simulink model "MODELODETURBINADERIO2017a"  (R2017a)
settings: Solver=FixedStepAuto  StartTime=0.0  StopTime=500  FixedStep=50e-3  RelTol=1e-3
values from neighbouring files (symbols this model uses):
  A = pi()*((D/2)^2)    [MODELOHIDRO.m]    (also in MODELOHIDROV10.m; MODELOHIDROV2.m; MODELOHIDROV3.m; MODELOHIDROV4.m)
  a = 790.51    [MODELOHIDRO.m]    (also in MODELOHIDROV2.m; MODELOHIDROV3.m)
  B = 0    [MODELOHIDRO.m]    (also in MODELOHIDROV10.m; MODELOHIDROV2.m; MODELOHIDROV3.m; MODELOHIDROV4.m)
  b = 6900.50    (= 6900.5)    [MODELOHIDRO.m]    (also in MODELOHIDROV2.m; MODELOHIDROV3.m)
  Bi = 0.2287    [MODELOHIDRO.m]    (also in MODELOHIDROV10.m = 0.1; MODELOHIDROV2.m; MODELOHIDROV3.m; MODELOHIDROV4.m = 0.005)
  c = 23794    [MODELOHIDRO.m]    (also in MODELOHIDROV2.m; MODELOHIDROV3.m)
  D = 1    [MODELOHIDRO.m]    (also in MODELOHIDROV10.m; MODELOHIDROV2.m; MODELOHIDROV3.m; MODELOHIDROV4.m)
  d = 39268    [MODELOHIDRO.m]    (also in MODELOHIDROV2.m; MODELOHIDROV3.m)
  den = 1000    [MODELOHIDRO.m]    (also in MODELOHIDROV10.m; MODELOHIDROV2.m; MODELOHIDROV3.m; MODELOHIDROV4.m)
  e = 31863    [MODELOHIDRO.m]    (also in MODELOHIDROV2.m; MODELOHIDROV3.m)
  f = 10049    [MODELOHIDRO.m]    (also in MODELOHIDROV2.m; MODELOHIDROV3.m)
  FACTOR = 1/(2*pi())*60    [MODELOHIDRO.m]    (also in MODELOHIDROV2.m; MODELOHIDROV3.m)
  Ji = 1    [MODELOHIDRO.m]    (also in MODELOHIDROV10.m = 1.72; MODELOHIDROV2.m; MODELOHIDROV3.m; MODELOHIDROV4.m = 0.0465)
  k = 1    [MODELOHIDRO.m]    (also in MODELOHIDROV2.m; MODELOHIDROV3.m)
  Kb = 1.8    [MODELOHIDRO.m]    (also in MODELOHIDROV10.m = 6.2; MODELOHIDROV2.m; MODELOHIDROV3.m; MODELOHIDROV4.m = 0.027)
  Kp = 0.4    [MODELOHIDRO.m]    (also in MODELOHIDROV10.m = 5.6627; MODELOHIDROV2.m; MODELOHIDROV3.m; MODELOHIDROV4.m = 0.027)
  m = 5    [MODELOHIDRO.m]    (also in MODELOHIDROV2.m; MODELOHIDROV3.m)
  r = D/2    (= 0.5)    [MODELOHIDRO.m]    (also in MODELOHIDROV10.m; MODELOHIDROV2.m; MODELOHIDROV3.m; MODELOHIDROV4.m)
  Ri = 0.6    [MODELOHIDRO.m]    (also in MODELOHIDROV10.m = 0.973; MODELOHIDROV2.m; MODELOHIDROV3.m; MODELOHIDROV4.m = 1)
  T_d = 0    [MODELOHIDRO.m]    (also in MODELOHIDROV10.m; MODELOHIDROV2.m; MODELOHIDROV3.m; MODELOHIDROV4.m)
  z = 2    [MODELOHIDRO.m]    (also in MODELOHIDROV2.m; MODELOHIDROV3.m)
undefined symbols (not defined in the file or in its folder): sigbuilder_block
libraries: simulink x3
settings Model: Creator=zni.uao  LastModifiedBy=Hp 14
settings SimscapeCC: SimscapeNormalizeSystem=off

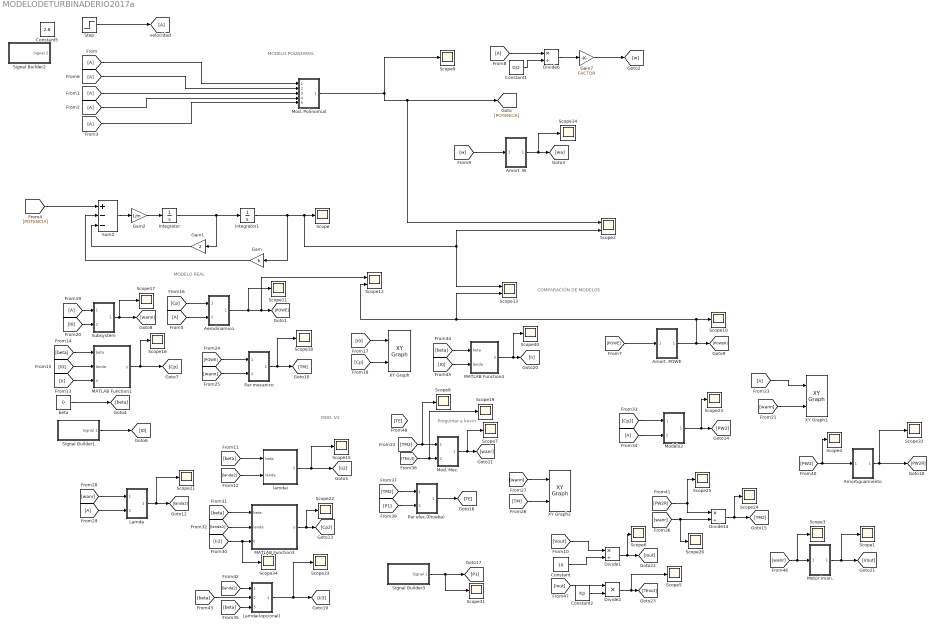
== system MODELODETURBINADERIO2017a ==
  note: MODELO POLINOMIAL
  note: MODELO REAL
  note: COMPARACIÓN DE MODELOS
  note: MOD. V2
  note: Preguntar a kevin
  Aerodinamico : Subsystem
  Amort. POWE : Subsystem
  Amort. W : Subsystem
  Amortiguamiento : Subsystem
  Constant : Constant  Value=10
  Constant1 : Constant  Value=D/2
  Constant2 : Constant  Value=Kp
  Constant5 : Constant  Value=2.8
  Divide1 : Product  Inputs=*/
  Divide14 : Product  Inputs=*/
  Divide2 : Product  Inputs=**
  Divide6 : Product  Inputs=*/
  Gain : Gain  Gain=k
  Gain1 : Gain  Gain=z
  Gain2 : Gain  Gain=1/m
  Gain7 : Gain  Gain=FACTOR
  Integrator : Integrator
  Integrator1 : Integrator
  Lamda : Subsystem
  Lamdai(opcional) : Subsystem
  MATLAB Function1 : MATLAB Function  TreatAsAtomicUnit=on
  MATLAB Function3 : MATLAB Function  TreatAsAtomicUnit=on
  MATLAB Function4 : MATLAB Function  TreatAsAtomicUnit=on
  Mod. Mec. : Subsystem
  Mod. Polinomial : Subsystem
  Modelo2 : Subsystem
  Motor iman. : Subsystem
  Par elec.(Prueba) : Subsystem
  Par mecanico : Subsystem
  Scope{,1,3..11,14..19,21..26,31..34,40} (28 alike) : Scope
  Scope12 : Scope  NumInputPorts=2
  Scope13 : Scope  NumInputPorts=2
  Scope2 : Scope  NumInputPorts=2
  Signal Builder1 : Subsystem  Tag=STV Subsys  LoadFcn=sigbuilder_block('load');  StartFcn=sigbuilder_block('start');  StopFcn=sigbuilder_block('stop');  ClipboardFcn=sigbuilder_block('clipboard');  mask(Sigbuilder block){tuvar=[0:10]}
      mask help: Simulink:masks:SigbuilderBlock_MD
      mask init:
      | if ~strcmp(get_param(bdroot(gcbh),'SimulationStatus'),'stopped') tuvar = sigbuilder_block('maskInit'); end
      settings: CopyFcn=sigbuilder_block('copy');  DeleteFcn=sigbuilder_block('delete');  ModelCloseFcn=sigbuilder_block('modelClose');  PreSaveFcn=sigbuilder_block('preSave');  PauseFcn=sigbuilder_block('pause');  ContinueFcn=sigbuilder_block('continue');  NameChangeFcn=sigbuilder_block('namechange');  OpenFcn=sigbuilder_block('open',[169.5 67.5 550.5 359.25 ]);  CloseFcn=sigbuilder_block('close');
      mask Display: plot(0, 0, 100, 100,[2, 2, 32, 32, 2], [68, 8, 8, 68, 68],[32, 2], [38, 38], [32, 19, 2],[53, 60, 44], [32, 17, 17, 2],[16, 16, 31, 31]);txt = getActiveGroup(gcbh);text(2, 100, txt,'verticalAlignment', 'top');
  Signal Builder2 : Subsystem  Tag=STV Subsys  LoadFcn=sigbuilder_block('load');  StartFcn=sigbuilder_block('start');  StopFcn=sigbuilder_block('stop');  ClipboardFcn=sigbuilder_block('clipboard');  mask(Sigbuilder block){tuvar=[0:10]}
      mask help: Simulink:masks:SigbuilderBlock_MD
      mask init:
      | if ~strcmp(get_param(bdroot(gcbh),'SimulationStatus'),'stopped') tuvar = sigbuilder_block('maskInit'); end
      settings: CopyFcn=sigbuilder_block('copy');  DeleteFcn=sigbuilder_block('delete');  ModelCloseFcn=sigbuilder_block('modelClose');  PreSaveFcn=sigbuilder_block('preSave');  PauseFcn=sigbuilder_block('pause');  ContinueFcn=sigbuilder_block('continue');  NameChangeFcn=sigbuilder_block('namechange');  OpenFcn=sigbuilder_block('open',[197.25 66 550.5 359.25 ]);  CloseFcn=sigbuilder_block('close');
      mask Display: plot(0, 0, 100, 100,[2, 2, 32, 32, 2], [68, 8, 8, 68, 68],[32, 2], [38, 38], [32, 19, 2],[53, 60, 44], [32, 17, 17, 2],[16, 16, 31, 31]);txt = getActiveGroup(gcbh);text(2, 100, txt,'verticalAlignment', 'top');
  Signal Builder3 : Subsystem  Tag=STV Subsys  LoadFcn=sigbuilder_block('load');  StartFcn=sigbuilder_block('start');  StopFcn=sigbuilder_block('stop');  ClipboardFcn=sigbuilder_block('clipboard');  mask(Sigbuilder block){tuvar=[0:10]}
      mask help: Simulink:masks:SigbuilderBlock_MD
      mask init:
      | if ~strcmp(get_param(bdroot(gcbh),'SimulationStatus'),'stopped') tuvar = sigbuilder_block('maskInit'); end
      settings: CopyFcn=sigbuilder_block('copy');  DeleteFcn=sigbuilder_block('delete');  ModelCloseFcn=sigbuilder_block('modelClose');  PreSaveFcn=sigbuilder_block('preSave');  PauseFcn=sigbuilder_block('pause');  ContinueFcn=sigbuilder_block('continue');  NameChangeFcn=sigbuilder_block('namechange');  OpenFcn=sigbuilder_block('open',[250.5 81.75 550.5 359.25 ]);  CloseFcn=sigbuilder_block('close');
      mask Display: plot(0, 0, 100, 100,[2, 2, 32, 32, 2], [68, 8, 8, 68, 68],[32, 2], [38, 38], [32, 19, 2],[53, 60, 44], [32, 17, 17, 2],[16, 16, 31, 31]);txt = getActiveGroup(gcbh);text(2, 100, txt,'verticalAlignment', 'top');
  Step : Step  Time=250  Before=2.5  After=2.888  SampleTime=0
  Subsystem : Subsystem
  Sum2 : Sum  Inputs=+--
  XY Graph : simulink/Sinks/XY Graph  xmin=1  xmax=20  ymin=0  ymax=0.56  st=0.1
  XY Graph1 : simulink/Sinks/XY Graph  xmin=1  xmax=20  ymin=0  ymax=0.56  st=0.1
  XY Graph2 : simulink/Sinks/XY Graph  xmin=1  xmax=20  ymin=0  ymax=0.56  st=0.1
  beta : Constant  Value=0
  lamdai : MATLAB Function  TreatAsAtomicUnit=on
  wires:
  Gain/1 -> Sum2/2
  Integrator1/1 -> Scope13/1, Scope2/2, Scope/1, Gain/1
  Gain1/1 -> Sum2/3
  Sum2/1 -> Gain2/1
  Gain2/1 -> Integrator/1
  [POTENCIA] -> Sum2/1
  Integrator/1 -> Gain1/1, Integrator1/1
  [A] -> Divide6/1
  Constant1/1 -> Divide6/2
  Divide6/1 -> Gain7/1
  Gain7/1 -> [w]
  beta/1 -> [beta]
  [Ii] -> MATLAB Function1/3(Ii)
  [beta] -> MATLAB Function1/1(beta)
  [I0] -> MATLAB Function1/2(landa)
  MATLAB Function1/1(y) -> Scope16/1, [Cp]
  [I0] -> XY Graph/1
  [wann] -> XY Graph1/2
  [A] -> XY Graph1/1
  [TM] -> XY Graph2/2
  [wann] -> XY Graph2/1
  MATLAB Function3/1(y) -> [Cp2], Scope22/1
  [beta] -> MATLAB Function3/1(beta)
  [landa2] -> MATLAB Function3/2(landa)
  [Ii2] -> Scope34/1, MATLAB Function3/3(Ii)
  Divide14/1 -> [TM2], Scope24/1
  [wanr] -> Scope26/1, Divide14/2
  [PW2R] -> Scope25/1, Divide14/1
  Signal Builder3/1(Signal 1) -> Scope31/1, [P1]
  [PW2] -> Amortiguamiento/1(In1), Scope4/1
  MATLAB Function4/1(Ii) -> Scope40/1, [Ii]
  [I0] -> MATLAB Function4/2(landa)
  [beta] -> MATLAB Function4/1(beta)
  lamdai/1(Ii) -> [Ii2], Scope15/1
  [landa2] -> lamdai/2(landa)
  [beta] -> lamdai/1(beta)
  Signal Builder1/1(Signal 1) -> [I0]
  Modelo2/1(Out1) -> Scope23/1, [PW2]
  [Cp2] -> Modelo2/1(In1)
  [A] -> Modelo2/2(In2)
  Par mecanico/1(Out1) -> [TM], Scope18/1
  [POWE] -> Par mecanico/1(In1)
  [wann] -> Par mecanico/2(In2)
  Aerodinamico/1(Out1) -> Scope11/1, Scope12/1, [POWE]
  [Cp] -> Aerodinamico/1(In1)
  [A] -> Aerodinamico/2(In2)
  [TM2] -> Par elec.(Prueba)/1(In1)
  [P1] -> Par elec.(Prueba)/2(In2)
  Par elec.(Prueba)/1(Out1) -> [TE]
  Lamda/1(Out1) -> [landa2], Scope21/1
  [wanr] -> Lamda/1(In1)
  [A] -> Lamda/2(In2)
  Lamdai(opcional)/1(Out1) -> Scope33/1, [Ii3]
  [landa2] -> Lamdai(opcional)/1(In1)
  [beta] -> Lamdai(opcional)/2(In2)
  [beta] -> Lamdai(opcional)/3(In3)
  [TM2] -> Scope8/1, Mod. Mec./1(In1)
  [TEout] -> Scope19/1, Mod. Mec./2(In2)
  Mod. Mec./1(Out1) -> Scope7/1, [wanr]
  [Cp] -> XY Graph/2
  Mod. Polinomial/1(Out1) -> Scope2/1, [POTENCIA], Scope9/1
  [A] -> Mod. Polinomial/1(In1)
  [A] -> Mod. Polinomial/2(In2)
  [A] -> Mod. Polinomial/3(In3)
  [A] -> Mod. Polinomial/4(In4)
  [A] -> Mod. Polinomial/5(In5)
  [wanr] -> Scope3/1, Motor iman./1(In1)
  Motor iman./1(Out1) -> Scope1/1, [Vout]
  Amortiguamiento/1(Out1) -> Scope32/1, [PW2R]
  Subsystem/1(Out1) -> [wann], Scope17/1
  [A] -> Subsystem/1(In1)
  [I0] -> Subsystem/2(In2)
  Amort. POWE/1(Out1) -> [POWER], Scope10/1, Scope12/2, Scope13/2
  [POWE] -> Amort. POWE/1(In1)
  [w] -> Amort. W/1(In1)
  Amort. W/1(Out1) -> Scope14/1, [wa]
  [Vout] -> Divide1/1
  Constant/1 -> Divide1/2
  Divide1/1 -> Scope6/1, [Iout]
  [Iout] -> Divide2/1
  Constant2/1 -> Divide2/2
  Divide2/1 -> Scope5/1, [TEout]
  Step/1 -> [A]

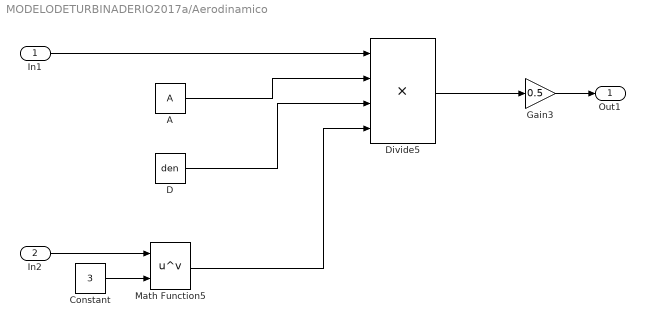
== system MODELODETURBINADERIO2017a/Aerodinamico ==
  In1 : Inport
  In2 : Inport  Port=2
  A : Constant  Value=A
  Constant : Constant  Value=3
  D : Constant  Value=den
  Divide5 : Product  Inputs=****  SaturateOnIntegerOverflow=on  RndMeth=Zero
  Gain3 : Gain  Gain=0.5
  Math Function5 : Math  Operator=pow  SaturateOnIntegerOverflow=on
  Out1 : Outport
  wires:
  Constant/1 -> Math Function5/2
  In2/1 -> Math Function5/1
  Math Function5/1 -> Divide5/4
  A/1 -> Divide5/2
  Divide5/1 -> Gain3/1
  D/1 -> Divide5/3
  In1/1 -> Divide5/1
  Gain3/1 -> Out1/1

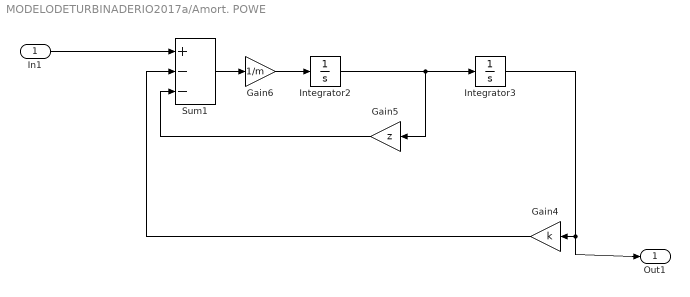
== system MODELODETURBINADERIO2017a/Amort. POWE ==
  In1 : Inport
  Gain4 : Gain  Gain=k
  Gain5 : Gain  Gain=z
  Gain6 : Gain  Gain=1/m
  Integrator2 : Integrator
  Integrator3 : Integrator
  Sum1 : Sum  Inputs=+--
  Out1 : Outport
  wires:
  Sum1/1 -> Gain6/1
  Integrator3/1 -> Out1/1, Gain4/1
  Gain4/1 -> Sum1/2
  Integrator2/1 -> Gain5/1, Integrator3/1
  Gain5/1 -> Sum1/3
  In1/1 -> Sum1/1
  Gain6/1 -> Integrator2/1

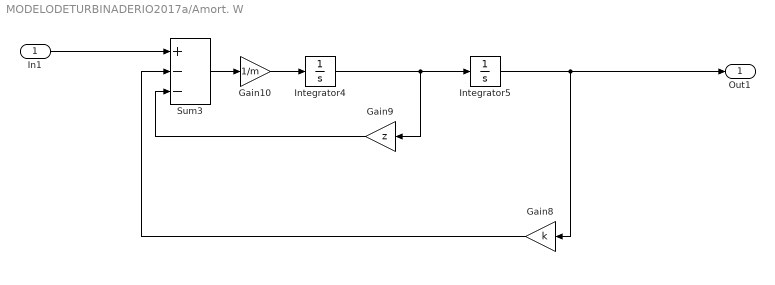
== system MODELODETURBINADERIO2017a/Amort. W ==
  In1 : Inport
  Gain10 : Gain  Gain=1/m
  Gain8 : Gain  Gain=k
  Gain9 : Gain  Gain=z
  Integrator4 : Integrator
  Integrator5 : Integrator
  Sum3 : Sum  Inputs=+--
  Out1 : Outport
  wires:
  In1/1 -> Sum3/1
  Gain9/1 -> Sum3/3
  Integrator4/1 -> Gain9/1, Integrator5/1
  Sum3/1 -> Gain10/1
  Integrator5/1 -> Out1/1, Gain8/1
  Gain10/1 -> Integrator4/1
  Gain8/1 -> Sum3/2

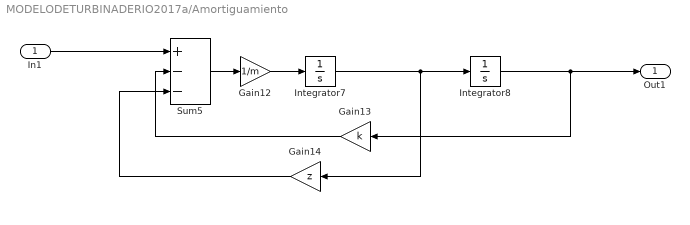
== system MODELODETURBINADERIO2017a/Amortiguamiento ==
  In1 : Inport
  Gain12 : Gain  Gain=1/m
  Gain13 : Gain  Gain=k
  Gain14 : Gain  Gain=z
  Integrator7 : Integrator
  Integrator8 : Integrator
  Sum5 : Sum  Inputs=+--
  Out1 : Outport
  wires:
  Gain13/1 -> Sum5/2
  Integrator8/1 -> Out1/1, Gain13/1
  Integrator7/1 -> Gain14/1, Integrator8/1
  Sum5/1 -> Gain12/1
  Gain12/1 -> Integrator7/1
  Gain14/1 -> Sum5/3
  In1/1 -> Sum5/1

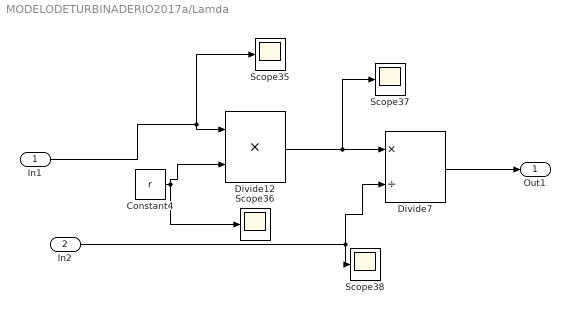
== system MODELODETURBINADERIO2017a/Lamda ==
  In1 : Inport
  In2 : Inport  Port=2
  Constant4 : Constant  Value=r
  Divide12 : Product  Inputs=**
  Divide7 : Product  Inputs=*/
  Scope{35..38} (4 alike) : Scope
  Out1 : Outport
  wires:
  Divide7/1 -> Out1/1
  In1/1 -> Divide12/1, Scope35/1
  Constant4/1 -> Divide12/2, Scope36/1
  In2/1 -> Divide7/2, Scope38/1
  Divide12/1 -> Scope37/1, Divide7/1

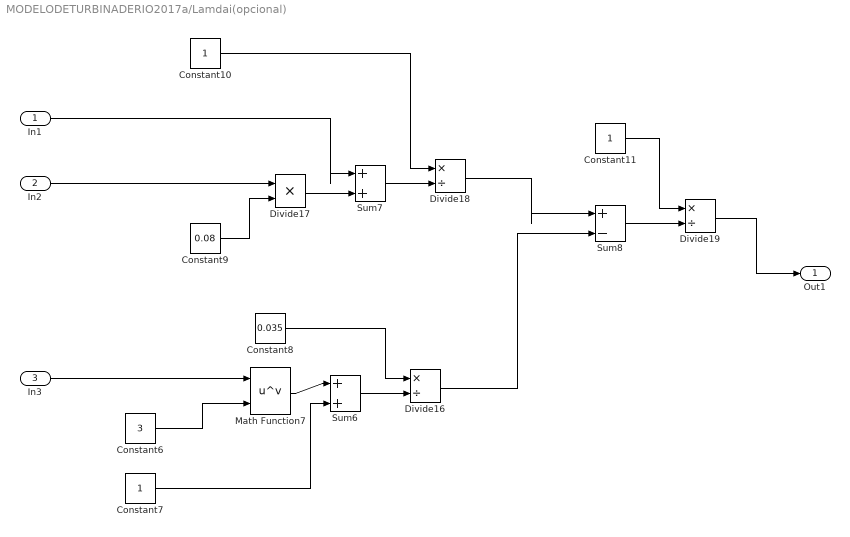
== system MODELODETURBINADERIO2017a/Lamdai(opcional) ==
  In1 : Inport
  In2 : Inport  Port=2
  In3 : Inport  Port=3
  Constant10 : Constant
  Constant11 : Constant
  Constant6 : Constant  Value=3
  Constant7 : Constant
  Constant8 : Constant  Value=0.035
  Constant9 : Constant  Value=0.08
  Divide16 : Product  Inputs=*/  SaturateOnIntegerOverflow=on  RndMeth=Zero
  Divide17 : Product  Inputs=**  SaturateOnIntegerOverflow=on  RndMeth=Zero
  Divide18 : Product  Inputs=*/  SaturateOnIntegerOverflow=on  RndMeth=Zero
  Divide19 : Product  Inputs=*/  SaturateOnIntegerOverflow=on  RndMeth=Zero
  Math Function7 : Math  Operator=pow  SaturateOnIntegerOverflow=on
  Sum6 : Sum  Inputs=|++
  Sum7 : Sum  Inputs=|++
  Sum8 : Sum  Inputs=|+-
  Out1 : Outport
  wires:
  Divide19/1 -> Out1/1
  Constant6/1 -> Math Function7/2
  Math Function7/1 -> Sum6/1
  Constant7/1 -> Sum6/2
  Sum6/1 -> Divide16/2
  In2/1 -> Divide17/1
  Constant8/1 -> Divide16/1
  Constant9/1 -> Divide17/2
  Divide17/1 -> Sum7/2
  In1/1 -> Sum7/1
  In3/1 -> Math Function7/1
  Sum8/1 -> Divide19/2
  Constant11/1 -> Divide19/1
  Constant10/1 -> Divide18/1
  Divide18/1 -> Sum8/1
  Sum7/1 -> Divide18/2
  Divide16/1 -> Sum8/2

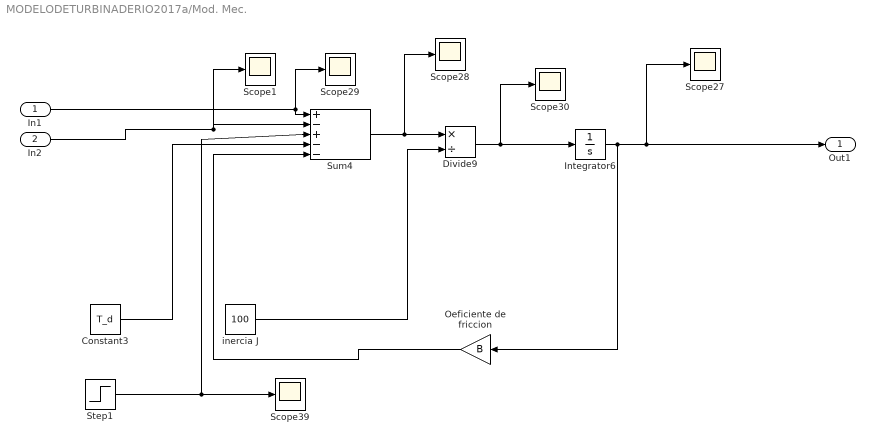
== system MODELODETURBINADERIO2017a/Mod. Mec. ==
  In1 : Inport
  In2 : Inport  Port=2
  Constant3 : Constant  Value=T_d
  Divide9 : Product  Inputs=*/
  Integrator6 : Integrator  InitialCondition=10
  Oeficiente de friccion : Gain  Gain=B
  Scope{1,27..30,39} (6 alike) : Scope
  Step1 : Step  Time=3  Before=5  After=0  SampleTime=0
  Sum4 : Sum  Inputs=|+-+--
  inercia J : Constant  Value=100
  Out1 : Outport
  wires:
  Oeficiente de friccion/1 -> Sum4/5
  Constant3/1 -> Sum4/4
  In2/1 -> Scope1/1, Sum4/2
  inercia J/1 -> Divide9/2
  Divide9/1 -> Scope30/1, Integrator6/1
  Sum4/1 -> Scope28/1, Divide9/1
  Integrator6/1 -> Out1/1, Scope27/1, Oeficiente de friccion/1
  In1/1 -> Scope29/1, Sum4/1
  Step1/1 -> Scope39/1, Sum4/3

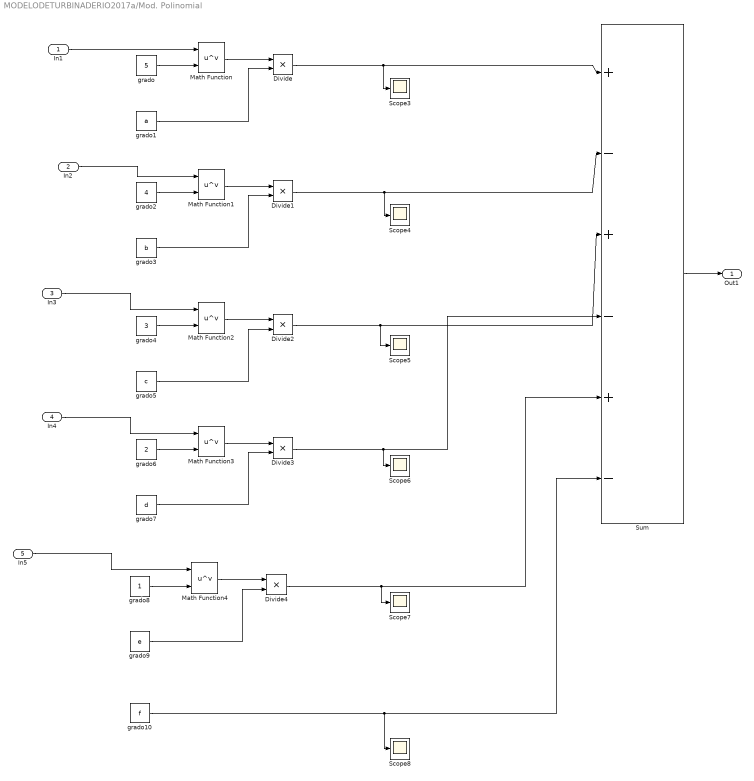
== system MODELODETURBINADERIO2017a/Mod. Polinomial ==
  In1 : Inport
  In2 : Inport  Port=2
  In3 : Inport  Port=3
  In4 : Inport  Port=4
  In5 : Inport  Port=5
  Divide{,1..4} (5 alike) : Product  Inputs=**
  Math Function{,1..4} (5 alike) : Math  Operator=pow  SaturateOnIntegerOverflow=on
  Scope{3..8} (6 alike) : Scope
  Sum : Sum  Inputs=|+-+-+-
  grado : Constant  Value=5
  grado1 : Constant  Value=a
  grado10 : Constant  Value=f
  grado2 : Constant  Value=4
  grado3 : Constant  Value=b
  grado4 : Constant  Value=3
  grado5 : Constant  Value=c
  grado6 : Constant  Value=2
  grado7 : Constant  Value=d
  grado8 : Constant
  grado9 : Constant  Value=e
  Out1 : Outport
  wires:
  In3/1 -> Math Function2/1
  Sum/1 -> Out1/1
  grado/1 -> Math Function/2
  grado9/1 -> Divide4/2
  grado3/1 -> Divide1/2
  In1/1 -> Math Function/1
  Math Function/1 -> Divide/1
  Divide2/1 -> Sum/3, Scope5/1
  grado2/1 -> Math Function1/2
  grado7/1 -> Divide3/2
  Divide3/1 -> Scope6/1, Sum/4
  grado10/1 -> Scope8/1, Sum/6
  Math Function3/1 -> Divide3/1
  Divide4/1 -> Scope7/1, Sum/5
  In2/1 -> Math Function1/1
  grado4/1 -> Math Function2/2
  Math Function1/1 -> Divide1/1
  grado1/1 -> Divide/2
  grado5/1 -> Divide2/2
  Math Function4/1 -> Divide4/1
  Divide/1 -> Scope3/1, Sum/1
  Math Function2/1 -> Divide2/1
  Divide1/1 -> Scope4/1, Sum/2
  In5/1 -> Math Function4/1
  In4/1 -> Math Function3/1
  grado6/1 -> Math Function3/2
  grado8/1 -> Math Function4/2

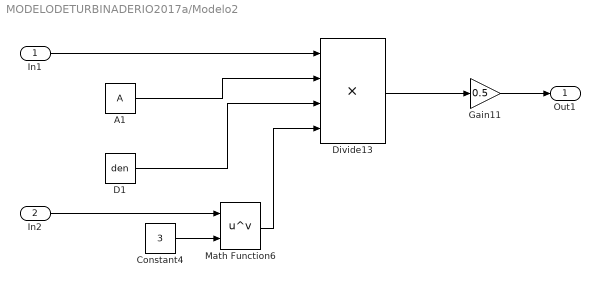
== system MODELODETURBINADERIO2017a/Modelo2 ==
  In1 : Inport
  In2 : Inport  Port=2
  A1 : Constant  Value=A
  Constant4 : Constant  Value=3
  D1 : Constant  Value=den
  Divide13 : Product  Inputs=****  SaturateOnIntegerOverflow=on  RndMeth=Zero
  Gain11 : Gain  Gain=0.5
  Math Function6 : Math  Operator=pow  SaturateOnIntegerOverflow=on
  Out1 : Outport
  wires:
  Constant4/1 -> Math Function6/2
  Divide13/1 -> Gain11/1
  D1/1 -> Divide13/3
  In1/1 -> Divide13/1
  Gain11/1 -> Out1/1
  A1/1 -> Divide13/2
  In2/1 -> Math Function6/1
  Math Function6/1 -> Divide13/4

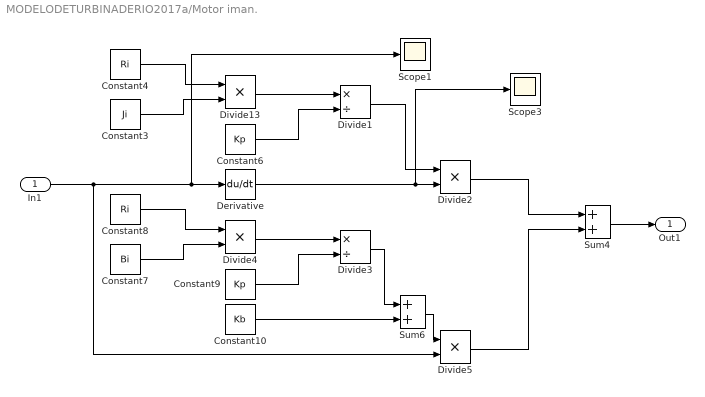
== system MODELODETURBINADERIO2017a/Motor iman. ==
  In1 : Inport
  Constant10 : Constant  Value=Kb
  Constant3 : Constant  Value=Ji
  Constant4 : Constant  Value=Ri
  Constant6 : Constant  Value=Kp
  Constant7 : Constant  Value=Bi
  Constant8 : Constant  Value=Ri
  Constant9 : Constant  Value=Kp
  Derivative : Derivative
  Divide1 : Product  Inputs=*/  SaturateOnIntegerOverflow=on  RndMeth=Zero
  Divide{2,4..5,13} (4 alike) : Product  Inputs=**  SaturateOnIntegerOverflow=on  RndMeth=Zero
  Divide3 : Product  Inputs=*/  SaturateOnIntegerOverflow=on  RndMeth=Zero
  Scope1 : Scope
  Scope3 : Scope
  Sum4 : Sum
  Sum6 : Sum
  Out1 : Outport
  wires:
  Constant10/1 -> Sum6/2
  Divide2/1 -> Sum4/1
  In1/1 -> Divide5/2, Scope1/1, Derivative/1
  Divide3/1 -> Sum6/1
  Divide13/1 -> Divide1/1
  Constant6/1 -> Divide1/2
  Constant4/1 -> Divide13/1
  Sum6/1 -> Divide5/1
  Divide1/1 -> Divide2/1
  Constant3/1 -> Divide13/2
  Constant9/1 -> Divide3/2
  Divide4/1 -> Divide3/1
  Constant7/1 -> Divide4/2
  Constant8/1 -> Divide4/1
  Derivative/1 -> Scope3/1, Divide2/2
  Sum4/1 -> Out1/1
  Divide5/1 -> Sum4/2

== system MODELODETURBINADERIO2017a/Par elec.(Prueba) ==
  In1 : Inport
  In2 : Inport  Port=2
  Divide15 : Product  Inputs=**
  Out1 : Outport
  wires:
  Divide15/1 -> Out1/1
  In2/1 -> Divide15/2
  In1/1 -> Divide15/1

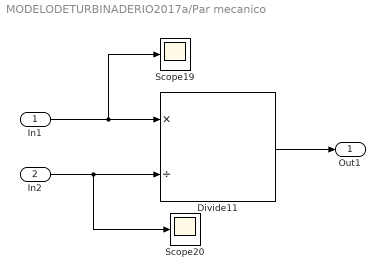
== system MODELODETURBINADERIO2017a/Par mecanico ==
  In1 : Inport
  In2 : Inport  Port=2
  Divide11 : Product  Inputs=*/
  Scope19 : Scope
  Scope20 : Scope
  Out1 : Outport
  wires:
  Divide11/1 -> Out1/1
  In2/1 -> Scope20/1, Divide11/2
  In1/1 -> Scope19/1, Divide11/1

== system MODELODETURBINADERIO2017a/Signal Builder1 ==
  Demux : Demux  Tag=STV Demux  Outputs=1
  FromWs : FromWorkspace  Tag=STV FromWs  VariableName=tuvar  SampleTime=0
      SigBuilderData=|
      | common.afterFinalStr = 'Extrapolate'
      | common.sampleTime = 0
      | dataSet.timeRange = [0 10]
      | dataSet.name = 'Group 1'
      | sbobj.Groups.Name = 'Group 1'
      | sbobj.Groups.Signals.Name = 'Signal 1'
      | sbobj.Groups.Signals.XData = [0 10]
      | sbobj.Groups.Signals.YData = [1 12]
  Signal 1 : Outport  Tag=STV Outport
  wires:
  FromWs/1 -> Demux/1
  Demux/1 -> Signal 1/1

== system MODELODETURBINADERIO2017a/Signal Builder2 ==
  Demux : Demux  Tag=STV Demux  Outputs=1
  FromWs : FromWorkspace  Tag=STV FromWs  VariableName=tuvar  SampleTime=0
      SigBuilderData=|
      | common.afterFinalStr = 'Extrapolate'
      | common.sampleTime = 0
      | dataSet.timeRange = [0 10]
      | dataSet.name = 'Group 1'
      | sbobj.Groups.Name = 'Group 1'
      | sbobj.Groups.Signals.Name = 'Signal 2'
      | sbobj.Groups.Signals.XData = [0 3 4 5 7 10]
      | sbobj.Groups.Signals.YData = [0 2 2 2.5 2.5 2.5]
  Signal 2 : Outport  Tag=STV Outport
  wires:
  FromWs/1 -> Demux/1
  Demux/1 -> Signal 2/1

== system MODELODETURBINADERIO2017a/Signal Builder3 ==
  Demux : Demux  Tag=STV Demux  Outputs=1
  FromWs : FromWorkspace  Tag=STV FromWs  VariableName=tuvar  SampleTime=0
      SigBuilderData=|
      | common.afterFinalStr = 'Extrapolate'
      | common.sampleTime = 0
      | dataSet.timeRange = [0 500]
      | dataSet.name = 'Group 1'
      | sbobj.Groups.Name = 'Group 1'
      | sbobj.Groups.Signals.Name = 'Signal 1'
      | sbobj.Groups.Signals.XData = [0 97 97 500]
      | sbobj.Groups.Signals.YData = [0 0.005 1 1]
      | sbobj.Groups.TimeRange = [0 500]
  Signal 1 : Outport  Tag=STV Outport
  wires:
  FromWs/1 -> Demux/1
  Demux/1 -> Signal 1/1

== system MODELODETURBINADERIO2017a/Subsystem ==
  In1 : Inport
  In2 : Inport  Port=2
  Constant2 : Constant  Value=r
  Divide10 : Product  Inputs=**
  Divide8 : Product  Inputs=*/
  Out1 : Outport
  wires:
  Divide8/1 -> Divide10/1
  In2/1 -> Divide10/2
  Divide10/1 -> Out1/1
  Constant2/1 -> Divide8/2
  In1/1 -> Divide8/1

== matlab function MODELODETURBINADERIO2017a/MATLAB Function1 ==
  data: beta input; y output; landa input; Ii input
function y = fcn(beta, landa,Ii)
w=0.5176; 
w1=116/Ii;
 w2=0.4*beta;
 w3=exp(-21/Ii);
 
 cp=w*(w1-w2-5)*w3+0.0068*landa;
 
 
 
 
 
y=cp;

== matlab function MODELODETURBINADERIO2017a/MATLAB Function3 ==
  data: beta input; y output; landa input; Ii input
function y = fcn(beta, landa,Ii)
w=0.5176; 
w1=116/Ii;
 w2=0.4*beta;
 w3=exp(-21/Ii);
 
 cp=w*(w1-w2-5)*w3+0.0068*landa;
 
 
 
 
 
y=cp;

== matlab function MODELODETURBINADERIO2017a/lamdai ==
  data: beta input; Ii output; landa input
function Ii = fcn(beta,landa)


Iii=(1/((landa+(0.08*beta))))-((0.035)/((beta^3)+1));
Ii=1/Iii;

== matlab function MODELODETURBINADERIO2017a/MATLAB Function4 ==
  data: beta input; Ii output; landa input
function Ii = fcn(beta,landa)


Iii=(1/((landa+(0.08*beta))))-((0.035)/((beta^3)+1));
Ii=1/Iii;
